simulink model "testChamberStability"  (R2023b)
settings: Solver=VariableStepAuto  StartTime=0.0  StopTime=32000  MaxStep=0.01  MinStep=0.001  RelTol=1e-3
libraries: slident x3
settings Model: Creator=hdt  LastModifiedBy=hdt
settings SolverCC: AutoInsertRateTranBlk=on

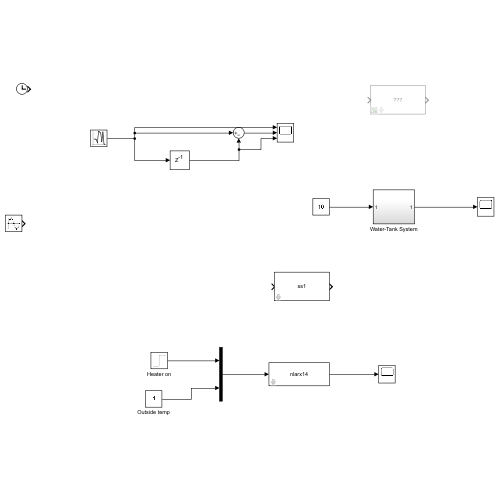
[thumbnail: Simulink's stored preview of the top-level diagram]
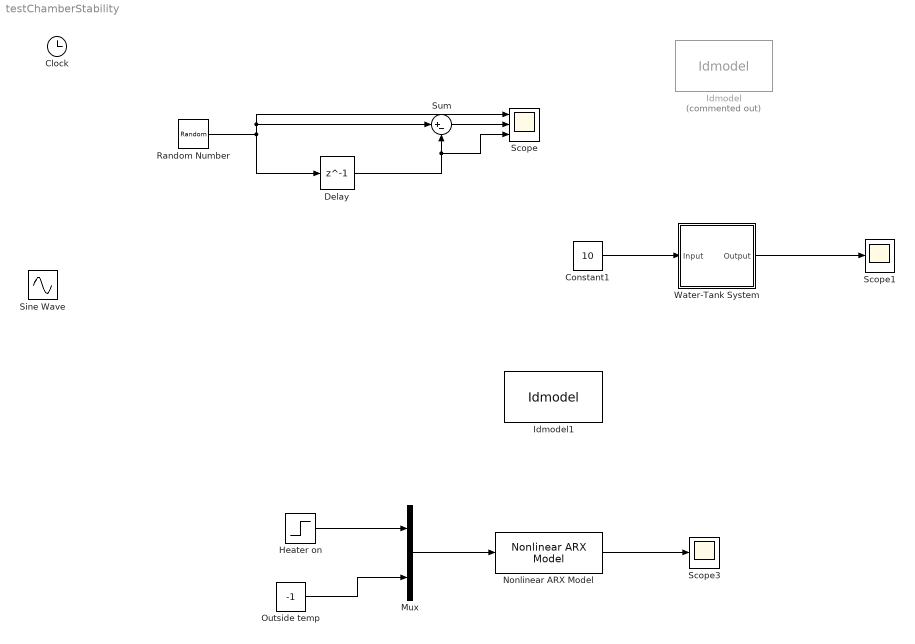
== system testChamberStability ==
  Clock : Clock
  Constant1 : Constant  Value=10
  Delay : Delay  DelayLength=1  SampleTime=1
  Heater on : Step  After=0  SampleTime=0
  Idmodel : slident/Models/Idmodel  Commented=on  sys=chamber  IC=0  noi=off  seed=[]
  Idmodel1 : slident/Models/Idmodel  sys=ss1  IC=[22.5; 22; -6]  noi=on  seed=[]
  Mux : Mux  Inputs=2
  Nonlinear ARX Model : slident/Models/Nonlinear ARX Model  sys=nlarx14  ICspec=Input and output values  X0=0  U0=[0; 10]  Y0=[23;22]
  Outside temp : Constant  Value=-1
  Random Number : RandomNumber  Seed=1  SampleTime=1
  Scope : Scope  NumInputPorts=3
  Scope1 : Scope
  Scope3 : Scope
  Sine Wave : Sin  SineType=Sample based  Samples=20  SampleTime=1
  Sum : Sum  Inputs=|+-
  Water-Tank System : Subsystem
  wires:
  Delay/1 -> Scope/3, Sum/2
  Sum/1 -> Scope/2
  Random Number/1 -> Sum/1, Scope/1, Delay/1
  Water-Tank System/1(Output) -> Scope1/1
  Heater on/1 -> Mux/1
  Constant1/1 -> Water-Tank System/1(Input)
  Mux/1 -> Nonlinear ARX Model/1
  Outside temp/1 -> Mux/2
  Nonlinear ARX Model/1 -> Scope3/1

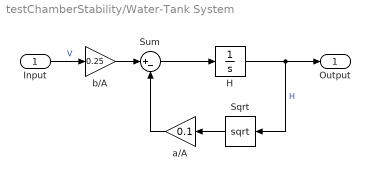
== system testChamberStability/Water-Tank System ==
  Input : Inport
  H : Integrator  InitialCondition=7.72065  LimitOutput=on  LowerSaturationLimit=0
  Sqrt : Sqrt  OutputSignalType=real
  Sum : Sum  Inputs=|+-  SaturateOnIntegerOverflow=on
  a/A : Gain  Gain=0.1  SaturateOnIntegerOverflow=on  OutDataTypeStr=Inherit: Same as input  ParamDataTypeStr=Inherit: Same as input
  b/A : Gain  Gain=0.25  SaturateOnIntegerOverflow=on  OutDataTypeStr=Inherit: Same as input  ParamDataTypeStr=Inherit: Same as input
  Output : Outport  VectorParamsAs1DForOutWhenUnconnected=off
  wires:
  b/A/1 -> Sum/1
  Sum/1 -> H/1
  H/1 -> Sqrt/1, Output/1  "H"
  Sqrt/1 -> a/A/1
  a/A/1 -> Sum/2
  Input/1 -> b/A/1  "V"
